simulink model "twoUpCnt"  (R2025b)
settings: Solver=FixedStepDiscrete  StartTime=0.0  StopTime=Inf  RelTol=1e-3
settings Model: Creator=Soochan Kim  LastModifiedBy=Soochan Kim
settings OptimizationCC: BlockReduction=off  ConditionallyExecuteInputs=off  DefaultParameterBehavior=Inlined
settings DebuggingCC: AlgebraicLoopMsg=error
settings HardwareCC: ProdBitPerPointer=32.0  ProdBitPerSizeT=32.0  ProdBitPerPtrDiffT=32.0  ProdLargestAtomicFloat=None  ProdIntDivRoundTo=Undefined  ProdEndianess=Unspecified  ProdWordSize=32.0  ProdHWDeviceType=ASIC/FPGA->ASIC/FPGA  TargetBitPerPointer=64.0  TargetBitPerSizeT=64.0  TargetBitPerPtrDiffT=64.0  TargetLongLongMode=on  TargetIntDivRoundTo=Zero  TargetEndianess=LittleEndian  TargetWordSize=64.0  TargetHWDeviceType=Custom Processor->MATLAB Host Computer  ProdEqTarget=off

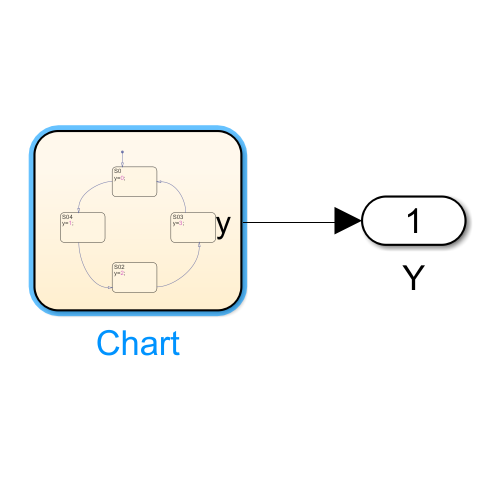
[thumbnail: Simulink's stored preview of the top-level diagram]
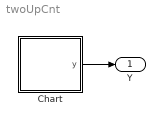
== system twoUpCnt ==
  Chart : Stateflow chart  TreatAsAtomicUnit=on
  Y : Outport
  wires:
  Chart/1(y) -> Y/1

== stateflow chart twoUpCnt/Chart ==
  settings: updateMethod=DISCRETE  stateMachineType=MOORE_MACHINE  executeAtInitialization=1  initializeOutput=1
  state S0
    y=uint8(0);
  state S1
    y=uint8(1);
  state S3
    y=uint8(3);
  state S2
    y=uint8(2);
  (default) -> S0
  S3 -> S0
  S0 -> S1
  S1 -> S2
  S2 -> S3
  data: y output uint8
